simulink model "trapezoidal_generator_converter_LCfilter"  (R2024b)
settings: Solver=VariableStepAuto  StartTime=0.0  StopTime=0.5  MaxStep=1e-6  RelTol=1e-3
libraries: spsMosfetLib x6, spsVoltageMeasurementLib x4, spsControlledVoltageSourceLib x3, spsSeriesRLCBranchLib x2, spsCurrentMeasurementLib x1, spsGroundLib x1, spsParallelRLCBranchLib x1, SignalEditorBlockLib x1, sps_lib x1, simulink x1
settings Model: Creator=byrin  LastModifiedBy=byrin
settings SolverCC: InitialStep=1e-7

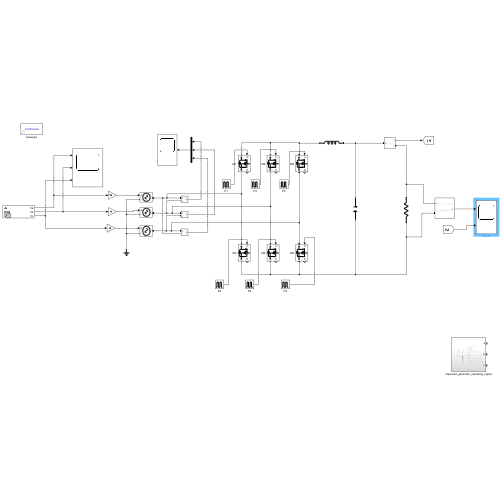
[thumbnail: Simulink's stored preview of the top-level diagram]
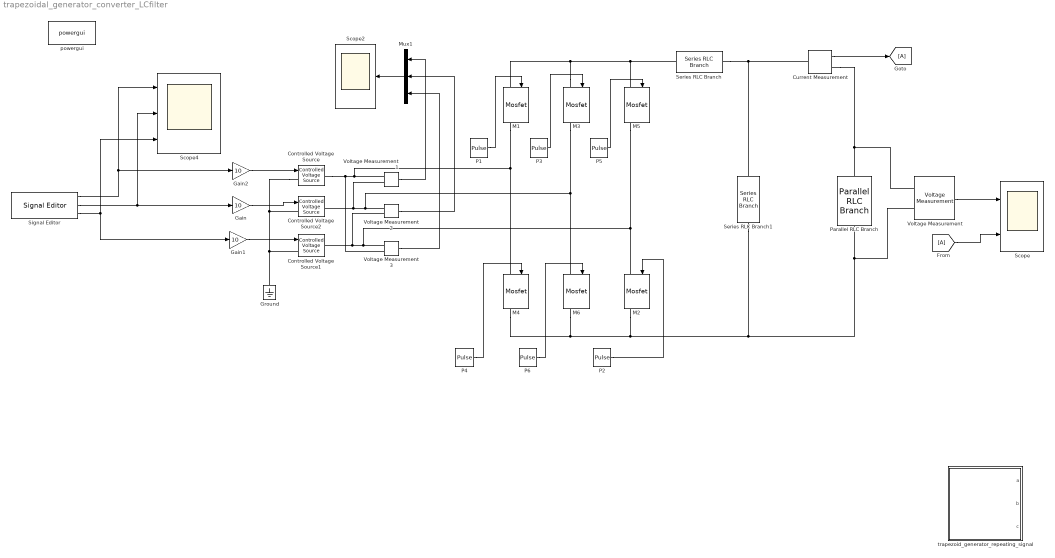
== system trapezoidal_generator_converter_LCfilter ==
  Controlled Voltage Source : spsControlledVoltageSourceLib/Controlled Voltage Source  Initialize=on  Source_Type=AC  Amplitude=120  Phase=0  Frequency=0  Measurements=None
  Controlled Voltage Source1 : spsControlledVoltageSourceLib/Controlled Voltage Source  Initialize=on  Source_Type=AC  Amplitude=120  Phase=120  Frequency=0  Measurements=None
  Controlled Voltage Source2 : spsControlledVoltageSourceLib/Controlled Voltage Source  Initialize=on  Source_Type=AC  Amplitude=120  Phase=-120  Frequency=0  Measurements=None
  Current Measurement : spsCurrentMeasurementLib/Current Measurement  PhasorSimulation=off  OutputType=Complex  PSBequivalent=0
  From : From
  Gain : Gain  Gain=10
  Gain1 : Gain  Gain=10
  Gain2 : Gain  Gain=10
  Goto : Goto
  Ground : spsGroundLib/Ground  LConnTagsString=a
  M{1..6} (6 alike) : spsMosfetLib/Mosfet  Ron=0.1  Lon=0  Rd=0.01  Vfd=0  IC=0  Rs=1e5  Cs=inf  Measurements=on
  Mux1 : Mux  Inputs=3
  P1 : DiscretePulseGenerator  PulseType=Time based  Period=20e-3  PulseWidth=5  PhaseDelay=(20e-3/360)*(30)
  P2 : DiscretePulseGenerator  PulseType=Time based  Period=20e-3  PulseWidth=10  PhaseDelay=(20e-3/360)*(90)
  P3 : DiscretePulseGenerator  PulseType=Time based  Period=20e-3  PulseWidth=10  PhaseDelay=(20e-3/360)*(150)
  P4 : DiscretePulseGenerator  PulseType=Time based  Period=20e-3  PulseWidth=5  PhaseDelay=(20e-3/360)*(210)
  P5 : DiscretePulseGenerator  PulseType=Time based  Period=20e-3  PulseWidth=10  PhaseDelay=(20e-3/360)*(270)
  P6 : DiscretePulseGenerator  PulseType=Time based  Period=20e-3  PulseWidth=10  PhaseDelay=(20e-3/360)*(330)
  Parallel RLC Branch : spsParallelRLCBranchLib/Parallel RLC Branch  LConnTagsString=a  RConnTagsString=__new0  BranchType=R  Resistance=10  Inductance=100e-3  SetiL0=off  InitialCurrent=0  Capacitance=100e-3  Setx0=off  InitialVoltage=0  Measurements=None
  Scope : Scope  NumInputPorts=2
  Scope2 : Scope
  Scope4 : Scope  NumInputPorts=3
  Series RLC Branch : spsSeriesRLCBranchLib/Series RLC Branch  LConnTagsString=__new0  RConnTagsString=__new0  BranchType=L  Resistance=1  Inductance=85e-3  SetiL0=off  InitialCurrent=0  Capacitance=1e-6  Setx0=off  InitialVoltage=0  Measurements=None
  Series RLC Branch1 : spsSeriesRLCBranchLib/Series RLC Branch  LConnTagsString=__new0  RConnTagsString=__new0  BranchType=C  Resistance=1  Inductance=1e-3  SetiL0=off  InitialCurrent=0  Capacitance=470e-6  Setx0=off  InitialVoltage=0  Measurements=None
  Signal Editor : SignalEditorBlockLib/Signal Editor  FileName=trapezoidal_3phase.mat  ActiveScenario=ds  ActiveSignal=Vc  IsBus=off  OutputBusObjectStr=Bus: BusObject  SampleTime=0  ZeroCross=off  OutputAfterFinalValue=Setting to zero  Unit=V  PreserveSignalName=on  ApplySigPropsToAllScenarios=on  ApplySigPropsToAllSignals=off
  Voltage Measurement{,1..3} (4 alike) : spsVoltageMeasurementLib/Voltage Measurement  PhasorSimulation=off  OutputType=Complex  PSBequivalent=0
  powergui : sps_lib/powergui  Priority=1  SimulationMode=Continuous  SampleTime=50e-6  frequency=60  Iterations=50  frequencyindice=0  Pbase=100e6  ErrMax=1e-4  UnitsV=kV  UnitsW=MW  buscounter=0  FunctionMessages=off  echomessages=off  EnableUseOfTLC=off  CurrentSourceSwitches=off  DisableSnubberDevices=off  DisableRonSwitches=off  DisableVfSwitches=off  DisplayEquations=off  AutomaticDiscreteSolvers=off  SolverType=Tustin/Backward Euler (TBE)  Interpol=off  ExternalGateDelay=off  methode=off  Ts=100  x0status=blocks  SPID=on  SwTol=0  HookPort=off  NonlinearTolerance=1e-4  nMaxIteration=100  ContinueOnMaxIteration=off  RestoreLinks=warning  ResistiveCurrentMeasurement=off  Frange=[0:2:500]  Ylog=off  Xlog=on  ShowGrid=off  save=off  variable=ZData  structure=0  ZoomFFT=off  StartTime=0.0  cycles=1  DisplayStyle=1  fundamental=60  FreqAxis=off  MaxFrequency=1000  frequencyindicesteady=1  RmsSteady=1  display=off
  trapezoid_generator_repeating_signal : Subsystem
  wires:
  P2/1 -> M2/1
  P3/1 -> M3/1
  P1/1 -> M1/1
  P5/1 -> M5/1
  P4/1 -> M4/1
  P6/1 -> M6/1
  Voltage Measurement/1 -> Scope/1
  From/1 -> Scope/2
  Current Measurement/1 -> Goto/1
  Mux1/1 -> Scope2/1
  Signal Editor/2 -> Scope4/2, Gain/1
  Signal Editor/1 -> Scope4/1, Gain2/1
  Signal Editor/3 -> Gain1/1, Scope4/3
  Gain1/1 -> Controlled Voltage Source1/1
  Gain2/1 -> Controlled Voltage Source/1
  Gain/1 -> Controlled Voltage Source2/1
  Voltage Measurement1/1 -> Mux1/1
  Voltage Measurement2/1 -> Mux1/2
  Voltage Measurement3/1 -> Mux1/3
  connections:
  Voltage Measurement2/LConn1 -- M6/LConn1 -- M3/RConn1 -- Voltage Measurement1/LConn2 -- Controlled Voltage Source2/RConn1
  Voltage Measurement3/LConn1 -- M2/LConn1 -- M5/RConn1 -- Voltage Measurement2/LConn2 -- Controlled Voltage Source1/RConn1
  Controlled Voltage Source/RConn1 -- Voltage Measurement3/LConn2 -- M4/LConn1 -- M1/RConn1 -- Voltage Measurement1/LConn1
  Current Measurement/RConn1 -- Parallel RLC Branch/LConn1 -- Voltage Measurement/LConn1
  M6/RConn1 -- M4/RConn1 -- Voltage Measurement/LConn2 -- Parallel RLC Branch/RConn1 -- Series RLC Branch1/RConn1 -- M2/RConn1
  M3/LConn1 -- Series RLC Branch/LConn1 -- M5/LConn1 -- M1/LConn1
  Controlled Voltage Source/LConn1 -- Ground/LConn1 -- Controlled Voltage Source1/LConn1 -- Controlled Voltage Source2/LConn1
  Series RLC Branch/RConn1 -- Current Measurement/LConn1 -- Series RLC Branch1/LConn1

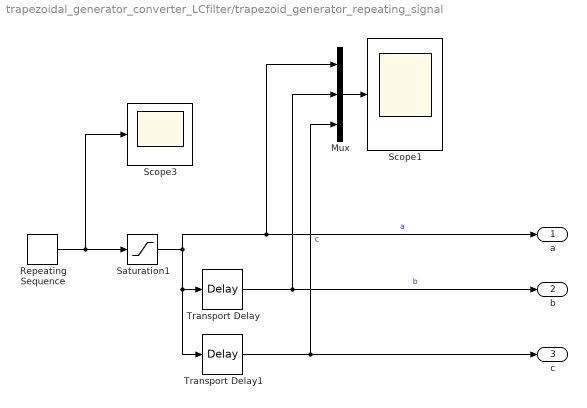
== system trapezoidal_generator_converter_LCfilter/trapezoid_generator_repeating_signal ==
  Mux : Mux  Inputs=3
  Repeating Sequence : simulink/Sources/Repeating Sequence  rep_seq_t=[0 0.005 0.01 0.015 0.02]  rep_seq_y=[0 1 0 -1 0 ]
  Saturation1 : Saturate
  Scope1 : Scope
  Scope3 : Scope
  Transport Delay : TransportDelay  DelayTime=(20e-3)*120/360
  Transport Delay1 : TransportDelay  DelayTime=(20e-3)*240/360
  a : Outport
  b : Outport  Port=2
  c : Outport  Port=3
  wires:
  Saturation1/1 -> a/1, Mux/1, Transport Delay1/1, Transport Delay/1  "a"
  Transport Delay1/1 -> c/1, Mux/3  "c"
  Repeating Sequence/1 -> Scope3/1, Saturation1/1
  Mux/1 -> Scope1/1
  Transport Delay/1 -> b/1, Mux/2  "b"
